simulink model "AnisoSM_ExtraSignalExcitation"  (R2019b)
settings: Solver=VariableStepAuto  StartTime=0.0  StopTime=10  RelTol=1e-3
undefined symbols (not defined in the file): DiscIntNeverNeededParam, Gamma_L, Gamma_R, init_value, LdRated, LqRated, psi_dh, psi_qh, PsiPMRated, RsRated, theta_error, TsimFSO, TsimMotor, Ud0, Udh, Uq0, Uqh, we
libraries: dsparch4 x4
settings Model: SimulationMode=accelerator  Creator=Downstream  LastModifiedBy=Downstream
settings DataIOCC: ReturnWorkspaceOutputs=off

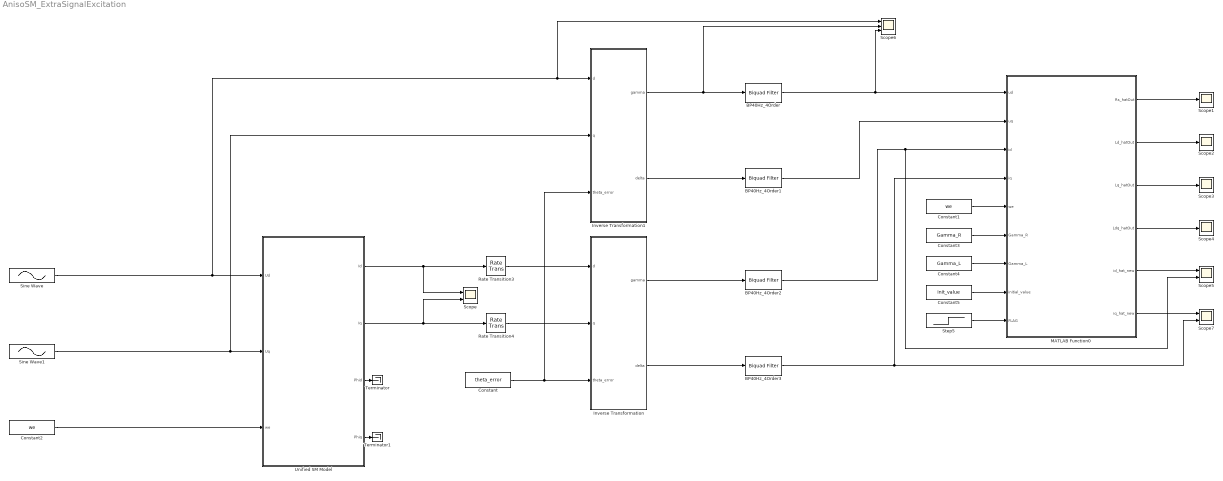
== system AnisoSM_ExtraSignalExcitation ==
  BP40Hz_4Order{,1..3} (4 alike) : dsparch4/Biquad Filter  Tag=BlockMethodSubSystem  FilterSource=Dialog parameters  CoeffSource=Specify via dialog  FilterObject=BQF  IIRFiltStruct=Direct form II  BiQuadCoeffs=[1 0 -1 1 -1.98869612032922305 0.989548115898122527;1 0 -1 1 -1.99235376140726217 0.992761680640966482]  ScaleValues=[0.00625541408694682902;0.00625541408694682902;1]  IC=0  ICnum=0  ICden=0  a0Flag=Warning  optimizeScaleValues=on  ScaleValueMode=Specify via input port (g)  InputProcessing=Columns as channels (frame based)  roundingMode=Floor  overflowMode=off  scaleValueFracLength=14  denProdOutputFracLength=30  denAccumFracLength=30  secondMemoryFracLength=15
      settings: SourceProductName=DSP System Toolbox
  Constant : Constant  Value=theta_error  SampleTime=TsimFSO
  Constant1 : Constant  Value=we  SampleTime=TsimFSO
  Constant2 : Constant  Value=we  SampleTime=TsimFSO
  Constant3 : Constant  Value=Gamma_R  SampleTime=TsimFSO
  Constant4 : Constant  Value=Gamma_L  SampleTime=TsimFSO
  Constant5 : Constant  Value=init_value  SampleTime=TsimFSO
  Inverse Transformation : Subsystem
  Inverse Transformation1 : Subsystem
  MATLAB Function0 : MATLAB Function  TreatAsAtomicUnit=on
  Rate Transition3 : RateTransition  OutPortSampleTime=TsimFSO
  Rate Transition4 : RateTransition  OutPortSampleTime=TsimFSO
  Scope : Scope  NumInputPorts=2
  Scope{1..4} (4 alike) : Scope
  Scope5 : Scope  NumInputPorts=2
  Scope6 : Scope  NumInputPorts=3
  Scope7 : Scope  NumInputPorts=2
  Sine Wave : Sin  Amplitude=Udh  Bias=Ud0  Frequency=40*2*pi  Phase=psi_dh  SampleTime=TsimFSO
  Sine Wave1 : Sin  Amplitude=Uqh  Bias=Uq0  Frequency=40*2*pi  Phase=psi_qh  SampleTime=TsimFSO
  Step5 : Step  Time=0.2  SampleTime=TsimFSO
  Terminator : Terminator
  Terminator1 : Terminator
  Unified SM Model : Subsystem
  wires:
  Unified SM Model/1(Id) -> Scope/1, Rate Transition3/1
  Unified SM Model/2(Iq) -> Scope/2, Rate Transition4/1
  Constant2/1 -> Unified SM Model/3(we)
  Sine Wave/1 -> Scope6/1, Inverse Transformation1/1(d), Unified SM Model/1(Ud)
  Sine Wave1/1 -> Inverse Transformation1/2(q), Unified SM Model/2(Uq)
  Unified SM Model/3(Phid) -> Terminator/1
  Unified SM Model/4(Phiq) -> Terminator1/1
  Constant/1 -> Inverse Transformation1/3(theta_error), Inverse Transformation/3(theta_error)
  Inverse Transformation/2(delta) -> BP40Hz_4Order3/1
  Inverse Transformation/1(gamma) -> BP40Hz_4Order2/1
  Inverse Transformation1/2(delta) -> BP40Hz_4Order1/1
  Inverse Transformation1/1(gamma) -> Scope6/2, BP40Hz_4Order/1
  BP40Hz_4Order/1 -> Scope6/3, MATLAB Function0/1(ud)
  BP40Hz_4Order1/1 -> MATLAB Function0/2(uq)
  Constant1/1 -> MATLAB Function0/5(we)
  Constant3/1 -> MATLAB Function0/6(Gamma_R)
  Constant4/1 -> MATLAB Function0/7(Gamma_L)
  Constant5/1 -> MATLAB Function0/8(initial_value)
  Step5/1 -> MATLAB Function0/9(FLAG)
  MATLAB Function0/1(Rs_hatOut) -> Scope1/1
  MATLAB Function0/2(Ld_hatOut) -> Scope2/1
  MATLAB Function0/3(Lq_hatOut) -> Scope3/1
  MATLAB Function0/4(Ldq_hatOut) -> Scope4/1
  MATLAB Function0/5(id_hat_new) -> Scope5/1
  BP40Hz_4Order2/1 -> MATLAB Function0/3(id), Scope5/2
  BP40Hz_4Order3/1 -> Scope7/2, MATLAB Function0/4(iq)
  Rate Transition3/1 -> Inverse Transformation/1(d)
  Rate Transition4/1 -> Inverse Transformation/2(q)
  MATLAB Function0/6(iq_hat_new) -> Scope7/1

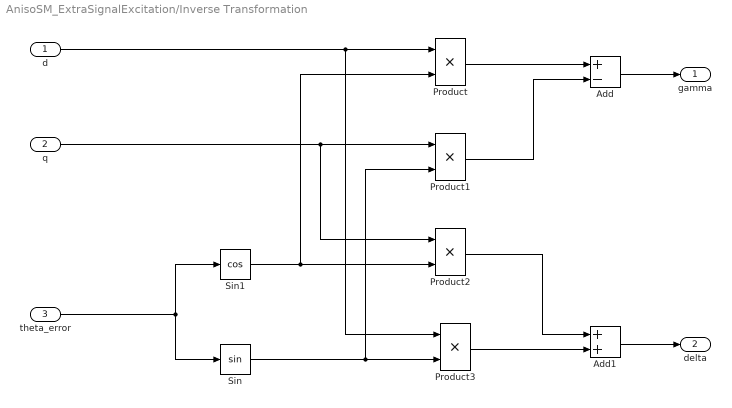
== system AnisoSM_ExtraSignalExcitation/Inverse Transformation ==
  d : Inport
  q : Inport  Port=2
  theta_error : Inport  Port=3
  Add : Sum  Inputs=+-
  Add1 : Sum
  Product{,1..3} (4 alike) : Product
  Sin : Trigonometry  OutputSignalType=real
  Sin1 : Trigonometry  Operator=cos  OutputSignalType=real
  gamma : Outport
  delta : Outport  Port=2
  wires:
  Product/1 -> Add/1
  Sin/1 -> Product3/2, Product1/2
  Product1/1 -> Add/2
  Add1/1 -> delta/1
  Sin1/1 -> Product2/2, Product/2
  Product2/1 -> Add1/1
  d/1 -> Product3/1, Product/1
  q/1 -> Product2/1, Product1/1
  Product3/1 -> Add1/2
  Add/1 -> gamma/1
  theta_error/1 -> Sin/1, Sin1/1

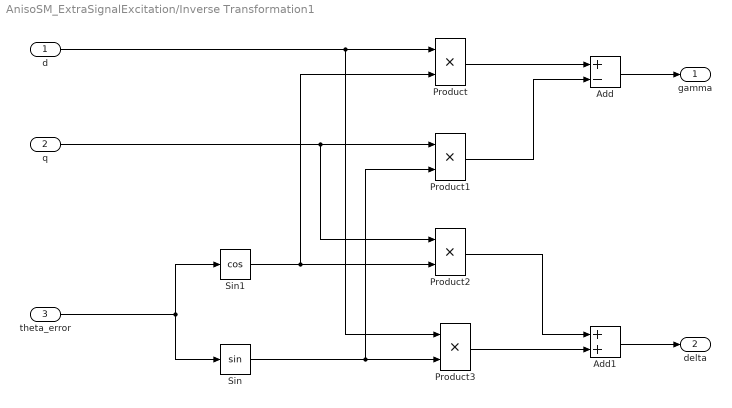
== system AnisoSM_ExtraSignalExcitation/Inverse Transformation1 ==
  d : Inport
  q : Inport  Port=2
  theta_error : Inport  Port=3
  Add : Sum  Inputs=+-
  Add1 : Sum
  Product{,1..3} (4 alike) : Product
  Sin : Trigonometry  OutputSignalType=real
  Sin1 : Trigonometry  Operator=cos  OutputSignalType=real
  gamma : Outport
  delta : Outport  Port=2
  wires:
  theta_error/1 -> Sin1/1, Sin/1
  Add/1 -> gamma/1
  Product3/1 -> Add1/2
  q/1 -> Product1/1, Product2/1
  d/1 -> Product/1, Product3/1
  Product2/1 -> Add1/1
  Sin1/1 -> Product/2, Product2/2
  Add1/1 -> delta/1
  Product1/1 -> Add/2
  Sin/1 -> Product1/2, Product3/2
  Product/1 -> Add/1

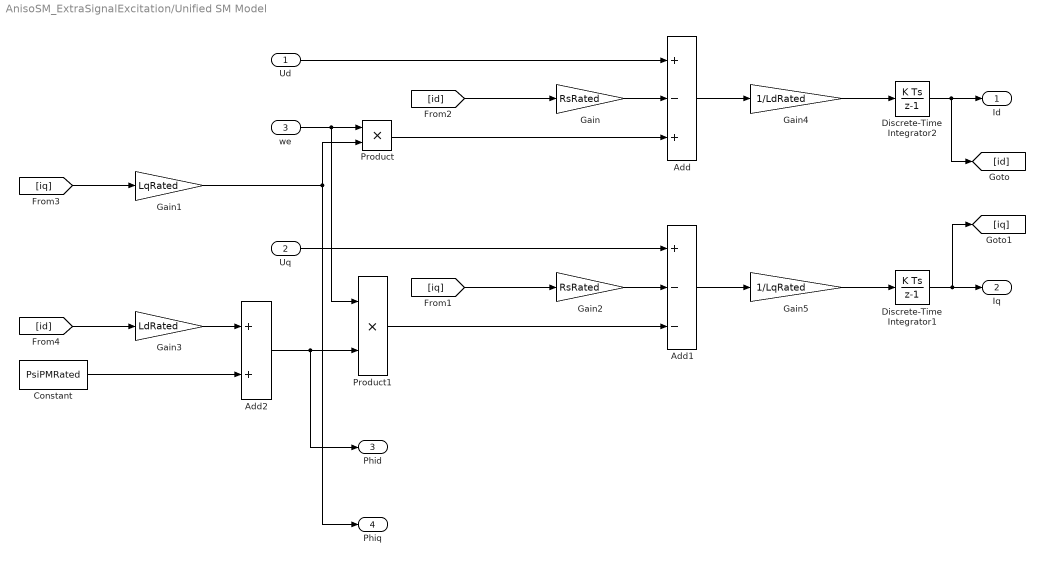
== system AnisoSM_ExtraSignalExcitation/Unified SM Model ==
  Ud : Inport
  Uq : Inport  Port=2
  we : Inport  Port=3
  Add : Sum  Inputs=+-+
  Add1 : Sum  Inputs=+--
  Add2 : Sum
  Constant : Constant  Value=PsiPMRated  SampleTime=TsimMotor
  Discrete-Time Integrator1 : DiscreteIntegrator  SampleTime=TsimMotor  UpperSaturationLimit=0  LowerSaturationLimit=-400  ICPrevOutput=DiscIntNeverNeededParam  ICPrevScaledInput=DiscIntNeverNeededParam
  Discrete-Time Integrator2 : DiscreteIntegrator  SampleTime=TsimMotor  UpperSaturationLimit=0  LowerSaturationLimit=-400  ICPrevOutput=DiscIntNeverNeededParam  ICPrevScaledInput=DiscIntNeverNeededParam
  Gain : Gain  Gain=RsRated
  Gain1 : Gain  Gain=LqRated
  Gain2 : Gain  Gain=RsRated
  Gain3 : Gain  Gain=LdRated
  Gain4 : Gain  Gain=1/LdRated
  Gain5 : Gain  Gain=1/LqRated
  Product : Product
  Product1 : Product
  Id : Outport
  Iq : Outport  Port=2
  Phid : Outport  Port=3
  Phiq : Outport  Port=4
  wires:
  Ud/1 -> Add/1
  we/1 -> Product/1, Product1/1
  Gain/1 -> Add/2
  [iq] -> Gain1/1
  [id] -> Gain/1
  Add/1 -> Gain4/1
  [id] -> Gain3/1
  [iq] -> Gain2/1
  Gain2/1 -> Add1/2
  Uq/1 -> Add1/1
  Gain3/1 -> Add2/1
  Constant/1 -> Add2/2
  Add2/1 -> Phid/1, Product1/2
  Product1/1 -> Add1/3
  Add1/1 -> Gain5/1
  Gain4/1 -> Discrete-Time Integrator2/1
  Gain5/1 -> Discrete-Time Integrator1/1
  Discrete-Time Integrator2/1 -> [id], Id/1
  Discrete-Time Integrator1/1 -> [iq], Iq/1
  Gain1/1 -> Phiq/1, Product/2
  Product/1 -> Add/3

== matlab function AnisoSM_ExtraSignalExcitation/MATLAB Function0 ==
  data: ud input; Rs_hatOut output; uq input; id input; iq input; we input; Ld_hatOut output; Lq_hatOut output; Ldq_hatOut output; id_hat_new output; iq_hat_new output; RsRated parameter; LqRated parameter; LdRated parameter; Gamma_R input; Gamma_L input; initial_value input; FLAG input
function [Rs_hatOut,Ld_hatOut,Lq_hatOut,Ldq_hatOut,id_hat_new,iq_hat_new] = MRAS_ParamId_HOT(ud,uq,id,iq,we,RsRated, LqRated, LdRated,Gamma_R,Gamma_L,initial_value,FLAG)
persistent id_hat iq_hat Rs_hat Ld_hat Lq_hat Ldq_hat;
if isempty(id_hat)
    id_hat = 0;
    iq_hat = 0;
    Rs_hat = RsRated*initial_value;
    Ld_hat = LdRated*initial_value;
    Lq_hat = LqRated*initial_value;
    Ldq_hat = 0;
end

    tilde_id = id_hat - id;
    tilde_iq = iq_hat - iq;
    u = [ud;uq];
    Tsim = 1e-4;
%     i = [id;iq];
    i_hat = [id_hat;iq_hat];
    L_hat = [Ld_hat Ldq_hat;Ldq_hat Lq_hat];
    J = [0 -1;1 0];
    I = [1 0;0  1];
    A = L_hat^-1 * (-Rs_hat * I - we * J * L_hat);
    B = L_hat^-1;
    Phi = I + A * Tsim + 0.5 * A^2 * Tsim^2 + 1/6 * A^3 * Tsim^3;
    G   = (Tsim * I + 0.5 * A * Tsim^2 + 1/6 * A^2 * Tsim^3 + 1/24 * A^3 * Tsim^4) * B;
%     Phi = I + A * Tsim;
%     G   = (Tsim * I) * B;
    i_hat_new = Phi * i_hat + G * u;
    id_hat_new = i_hat_new(1);
    iq_hat_new = i_hat_new(2);
    
    i_hat_dot = B * u + A * i_hat;
    if(FLAG == 1)
        dot_Rs_hat = (tilde_id * id_hat + tilde_iq * iq_hat) * Gamma_R;
        dot_Ld_hat =( we * id_hat * tilde_iq + tilde_id * i_hat_dot(1)) * Gamma_L;
        dot_Lq_hat =(-we * iq_hat * tilde_id + tilde_iq * i_hat_dot(2)) * Gamma_L;
        dot_Ldq_hat= Gamma_L * (0.5) * (-we * id_hat * tilde_id + we * iq_hat * tilde_iq + i_hat_dot(2) * tilde_id +i_hat_dot(1) * tilde_iq);
% dot_Ldq_hat = 0;
        %%%%%%%SPMSM Only%%%%%%%%%%%%
%         dot_Ld_hat = (dot_Ld_hat + dot_Lq_hat)/2;
%         dot_Lq_hat = dot_Ld_hat;
    else
        dot_Rs_hat = 0;
        dot_Ld_hat = 0;
        dot_Lq_hat = 0;
        dot_Ldq_hat = 0;
    end
        
    
    Ld_hat = Ld_hat + dot_Ld_hat * Tsim;% + 0.5 * Tsim^2 *dot_Ld_hat^2;
    Lq_hat = Lq_hat + dot_Lq_hat * Tsim;% + 0.5 * Tsim^2 *dot_Lq_hat^2;
    Ldq_hat = Ldq_hat + dot_Ldq_hat * Tsim;% + 0.5 * Tsim^2 *dot_Lq_hat^2;
    Rs_hat = Rs_hat + dot_Rs_hat * Tsim;% + 0.5 * Tsim^2 *dot_Rs_hat^2;
    if(Ld_hat > LdRated*2)
        Ld_hat = LdRated * 2;
    elseif(Ld_hat < LdRated*0.5)
        Ld_hat = LdRated * 0.5;
    end
    if(Lq_hat > LqRated*2)
        Lq_hat = LqRated * 2;
    elseif(Lq_hat < LqRated*0.5)
        Lq_hat = LqRated * 0.5;
    end
    if(Ldq_hat > (LqRated-LdRated))
        Ldq_hat = (LqRated-LdRated);
    elseif(Lq_hat < -(LqRated-LdRated))
        Ldq_hat = -(LqRated-LdRated);
    end
    
    if(Rs_hat > RsRated*2)
        Rs_hat = RsRated * 2;
    elseif(Rs_hat < RsRated*0.5)
        Rs_hat = RsRated * 0.5;
    end
    
    id_hat = id_hat_new;
    iq_hat = iq_hat_new;
    Rs_hatOut = Rs_hat;
    Ld_hatOut = Ld_hat;
    Lq_hatOut = Lq_hat;
    Ldq_hatOut = Ldq_hat;
end
